simulink model "lol"  (R2021b)
settings: Solver=FixedStepAuto  StartTime=0.0  StopTime=100  FixedStep=0.05  RelTol=1e-3
undefined symbols (not defined in the file or in its folder): DiscIntNeverNeededParam, Discrete, Time
libraries: simulink x1, ctrlSharedLib x1
settings Model: Creator=alunos_ar  LastModifiedBy=alunos_ar

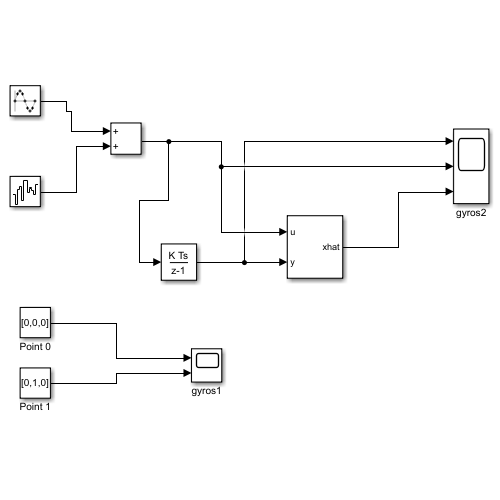
[thumbnail: Simulink's stored preview of the top-level diagram]
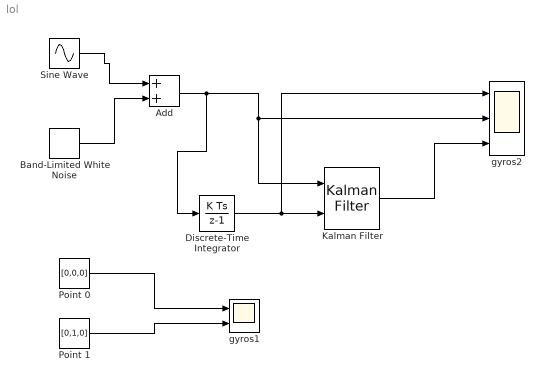
== system lol ==
  Add : Sum
  Band-Limited White Noise : simulink/Sources/Band-Limited White Noise  Cov=[10^(-3)]  Ts=0.05  seed=[23341]
  Discrete-Time Integrator : DiscreteIntegrator  SampleTime=-1  ICPrevOutput=DiscIntNeverNeededParam  ICPrevScaledInput=DiscIntNeverNeededParam
  Kalman Filter : ctrlSharedLib/Kalman Filter  TimeDomain=Discrete-Time  UseCurrentEstimator=on  ModelSource=LTI State-Space Variable  ModelSourceVariable=ss(0,1,1,0,0.05)  A=0.95  B=1  C=1  D=0  NumberOfStates=1  NumberOfInputs=1  NumberOfOutputs=1  InitialEstimateSource=Dialog  X0=0  P0=10  UseK=off  UseGH=off  NumberOfProcessNoiseInputs=1  G=1  TimeInvariantG=on  H=0  TimeInvariantH=on  Q=2  TimeInvariantQ=on  R=1  TimeInvariantR=on  N=0  TimeInvariantN=on  AddInputPort=on  AddEnablePort=off  OutputEstimatedY=off  OutputP=off  Ts=-1
  Point 0 : Constant  Value=[0,0,0]  VectorParams1D=off  SampleTime=-1
  Point 1 : Constant  Value=[0,1,0]
  Sine Wave : Sin  SineType=Sample based  Samples=100  SampleTime=0.05
  gyros1 : Scope  NumInputPorts=2
  gyros2 : Scope  NumInputPorts=3
  wires:
  Point 0/1 -> gyros1/1
  Point 1/1 -> gyros1/2
  Sine Wave/1 -> Add/1
  Band-Limited White Noise/1 -> Add/2
  Add/1 -> Discrete-Time Integrator/1, Kalman Filter/1, gyros2/2
  Kalman Filter/1 -> gyros2/3
  Discrete-Time Integrator/1 -> gyros2/1, Kalman Filter/2
